simulink model "Pedestrian_light"  (R2022a)
settings: Solver=FixedStepAuto  StartTime=0.0  StopTime=10000.0  FixedStep=1.0  RelTol=1e-3
settings Model: DataDictionary=TrafficLightComposer.sldd  Creator=Amin  LastModifiedBy=Amin

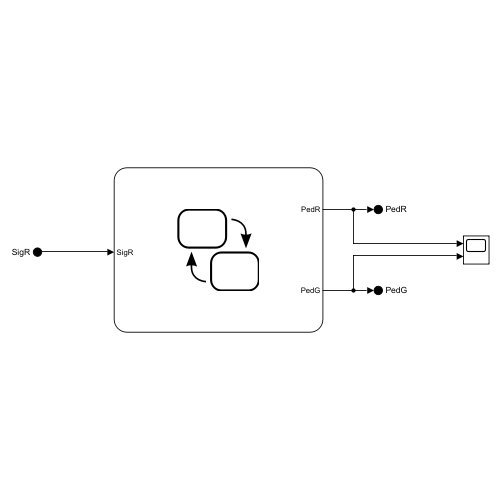
[thumbnail: Simulink's stored preview of the top-level diagram]
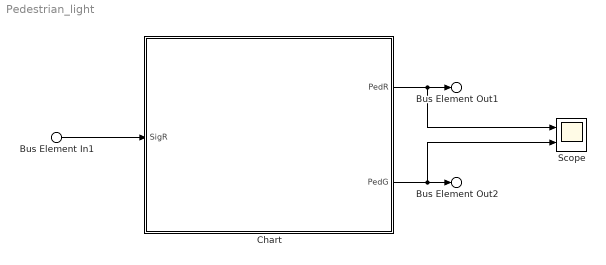
== system Pedestrian_light ==
  Bus Element In1 : Inport  PortName=SigR
  Chart : Stateflow chart  TreatAsAtomicUnit=on
  Scope : Scope  NumInputPorts=2
  Bus Element Out1 : Outport  PortName=PedR
  Bus Element Out2 : Outport  Port=2  PortName=PedG
  wires:
  Chart/2(PedG) -> Scope/2, Bus Element Out2/1
  Chart/1(PedR) -> Bus Element Out1/1, Scope/1
  Bus Element In1/1 -> Chart/1(SigR)

== stateflow chart Pedestrian_light/Chart ==
  state Green
  state Red
  Green -> Red [order 1] : [pcount>=60]{PedR=1;PedG=0}
  (default) -> Green : {pcount=0;PedG=1}
  Green -> Green [order 2] : {pcount=pcount+1;}
  Red -> Green : [SigR==1]{PedG=1;PedR=0;pcount=0;}
  data: SigR input boolean; PedR output; PedG output; pcount local
